simulink library "lib_Radiation_HeatXCoeffRefPlanar"  (R2015a)
settings: Solver=ode45  StartTime=0.0  StopTime=10.0  RelTol=1e-3
settings Model: Creator=jlkratz  LastModifiedBy=jlkratz

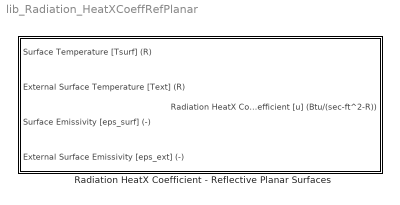
== system lib_Radiation_HeatXCoeffRefPlanar ==
  Radiation HeatX Coefficient - Reflective Planar Surfaces : Subsystem  mask(TSAT: Radiation HeatX Coefficient - Non-Reflective Sink Block){}
      mask help:
      | This function computes the radiation heat transfer coefficient when the radiation term is written in a linear form (q = u*(Text - Tsurf)). This block is applicable for radiation between two reflective parallel planar surfaces.
      |
      | Units are specified on the inport and outports so be sure to adhere to the appropriate units.
      mask Help: web(which('Radiation_TSAT_HeatXCoeffRefPlanar.html'),'-helpbrowser')

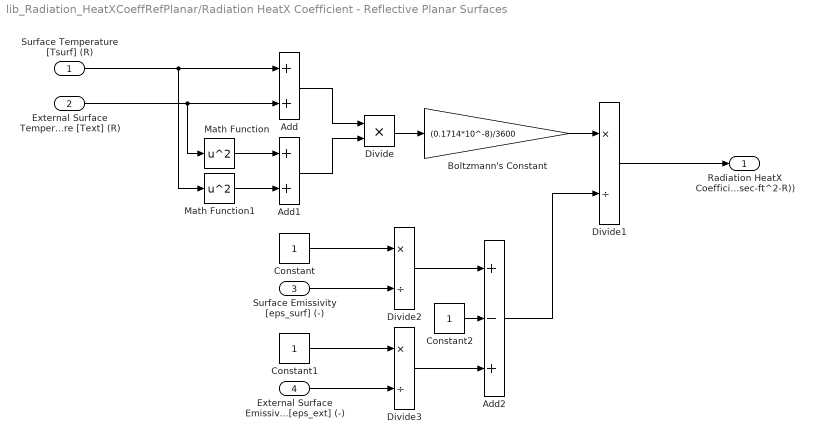
== system lib_Radiation_HeatXCoeffRefPlanar/Radiation HeatX Coefficient - Reflective Planar Surfaces ==
  Surface Temperature [Tsurf] (R) : Inport
  External Surface Temperature [Text] (R) : Inport  Port=2
  Surface Emissivity [eps_surf] (-) : Inport  Port=3
  External Surface Emissivity [eps_ext] (-) : Inport  Port=4
  Add : Sum
  Add1 : Sum
  Add2 : Sum  Inputs=+-+
  Boltzmann's Constant : Gain  Gain=(0.1714*10^-8)/3600
  Constant : Constant
  Constant1 : Constant
  Constant2 : Constant
  Divide : Product  Inputs=**
  Divide1 : Product  Inputs=*/
  Divide2 : Product  Inputs=*/
  Divide3 : Product  Inputs=*/
  Math Function : Math  Operator=square  SaturateOnIntegerOverflow=on
  Math Function1 : Math  Operator=square  SaturateOnIntegerOverflow=on
  Radiation HeatX Coefficient [u] (Btu/(sec-ft^2-R)) : Outport
  wires:
  Add2/1 -> Divide1/2
  Constant2/1 -> Add2/2
  Divide3/1 -> Add2/3
  Divide2/1 -> Add2/1
  External Surface Emissivity [eps_ext] (-)/1 -> Divide3/2
  Constant1/1 -> Divide3/1
  Surface Emissivity [eps_surf] (-)/1 -> Divide2/2
  Constant/1 -> Divide2/1
  Math Function1/1 -> Add1/2
  Divide1/1 -> Radiation HeatX Coefficient [u] (Btu/(sec-ft^2-R))/1
  Surface Temperature [Tsurf] (R)/1 -> Add/1, Math Function1/1
  External Surface Temperature [Text] (R)/1 -> Add/2, Math Function/1
  Divide/1 -> Boltzmann's Constant/1
  Add1/1 -> Divide/2
  Boltzmann's Constant/1 -> Divide1/1
  Add/1 -> Divide/1
  Math Function/1 -> Add1/1
